simulink model "Controller_PID"  (Simulink 8.9)
settings: Solver=ode1  StartTime=0.0  StopTime=5.12  FixedStep=0.001  RelTol=1e-3
values from neighbouring files (symbols this model uses):
  Acommands = DriveCommands(:,4)-HomePosDrive(4)    [MainContourControlExp.m]    (also in MainProgress.m = Pre_commands(4,:) - HomePosCommonds(4); MainProgress02.m = output_preditionnet(4,:) - HomePosCommonds(4))
  Ccommands = DriveCommands(:,5)-HomePosDrive(5)    [MainContourControlExp.m]    (also in MainProgress.m = Pre_commands(5,:) - HomePosCommonds(5); MainProgress02.m = output_preditionnet(5,:) - HomePosCommonds(5))
  PlantADen = [1 PlantAPara.a1 PlantAPara.a0]    [MainContourControlExp.m]    (also in MainProgress.m; MainProgress02.m)
  PlantANum = [PlantAPara.b1 PlantAPara.b0]    [MainContourControlExp.m]    (also in MainProgress.m; MainProgress02.m)
  PlantCDen = [1 PlantCPara.a1 PlantCPara.a0]    [MainContourControlExp.m]    (also in MainProgress.m; MainProgress02.m)
  PlantCNum = [PlantCPara.b1 PlantCPara.b0]    [MainContourControlExp.m]    (also in MainProgress.m; MainProgress02.m)
  PlantXDen = [1 PlantXPara.a1 PlantXPara.a0]    [MainContourControlExp.m]    (also in MainProgress.m; MainProgress02.m)
  PlantXNum = [PlantXPara.b1 PlantXPara.b0]    [MainContourControlExp.m]    (also in MainProgress.m; MainProgress02.m)
  PlantYDen = [1 PlantYPara.a1 PlantYPara.a0]    [MainContourControlExp.m]    (also in MainProgress.m; MainProgress02.m)
  PlantYNum = [PlantYPara.b1 PlantYPara.b0]    [MainContourControlExp.m]    (also in MainProgress.m; MainProgress02.m)
  PlantZDen = [1 PlantZPara.a1 PlantZPara.a0]    [MainContourControlExp.m]    (also in MainProgress.m; MainProgress02.m)
  PlantZNum = [PlantZPara.b1 PlantZPara.b0]    [MainContourControlExp.m]    (also in MainProgress.m; MainProgress02.m)
  Ts = 0.001    [MainContourControlExp.m]    (also in MainProgress.m; MainProgress02.m)
  Xcommands = DriveCommands(:,1)-HomePosDrive(1)    [MainContourControlExp.m]    (also in MainProgress.m = Pre_commands(1,:) - HomePosCommonds(1); MainProgress02.m = output_preditionnet(1,:) - HomePosCommonds(1))
  Ycommands = DriveCommands(:,2)-HomePosDrive(2)    [MainContourControlExp.m]    (also in MainProgress.m = Pre_commands(2,:) - HomePosCommonds(2); MainProgress02.m = output_preditionnet(2,:) - HomePosCommonds(2))
  Zcommands = DriveCommands(:,3)-HomePosDrive(3)    [MainContourControlExp.m]    (also in MainProgress.m = Pre_commands(3,:) - HomePosCommonds(3); MainProgress02.m = output_preditionnet(3,:) - HomePosCommonds(3))
undefined symbols (not defined in the file or in its folder): DiscIntNeverNeededParam
libraries: powerlib_extras x10, simulink x5
settings Model: SuppressorTable=22 serialization::archive 11 0 6 0 0 0 11 0  Creator=e308  LastModifiedBy=e308
settings DataIOCC: LimitDataPoints=off  SaveFormat=Dataset  SignalLoggingSaveFormat=Dataset
settings OptimizationCC: LifeSpan=auto
settings DebuggingCC: UnderspecifiedInitializationDetection=Simplified  MergeDetectMultiDrivingBlocksExec=error  FcnCallInpInsideContextMsg=error  StateNameClashWarn=none  SFUnexpectedBacktrackingDiag=error  SFNoUnconditionalDefaultTransitionDiag=error  SFExecutionAtInitializationDiag=warning
settings HardwareCC: ProdBitPerPointer=64  ProdBitPerSizeT=64  ProdBitPerPtrDiffT=64  ProdLargestAtomicFloat=Float  ProdIntDivRoundTo=Zero  ProdEndianess=LittleEndian  ProdWordSize=64  ProdHWDeviceType=Intel->x86-64 (Windows64)
settings ModelReferenceCC: PropagateSignalLabelsOutOfModel=on
settings GRTTargetCC: TargetLangStandard=C99 (ISO)  GeneratePreprocessorConditionals=Use local settings  CombineOutputUpdateFcns=on  GRTInterface=off
settings ConfigComp: CovMetricSettings=dwe  CovHtmlReporting=off  CovSaveCumulativeToWorkspaceVar=off  CovSaveSingleToWorkspaceVar=off  CovExternalEMLEnable=on

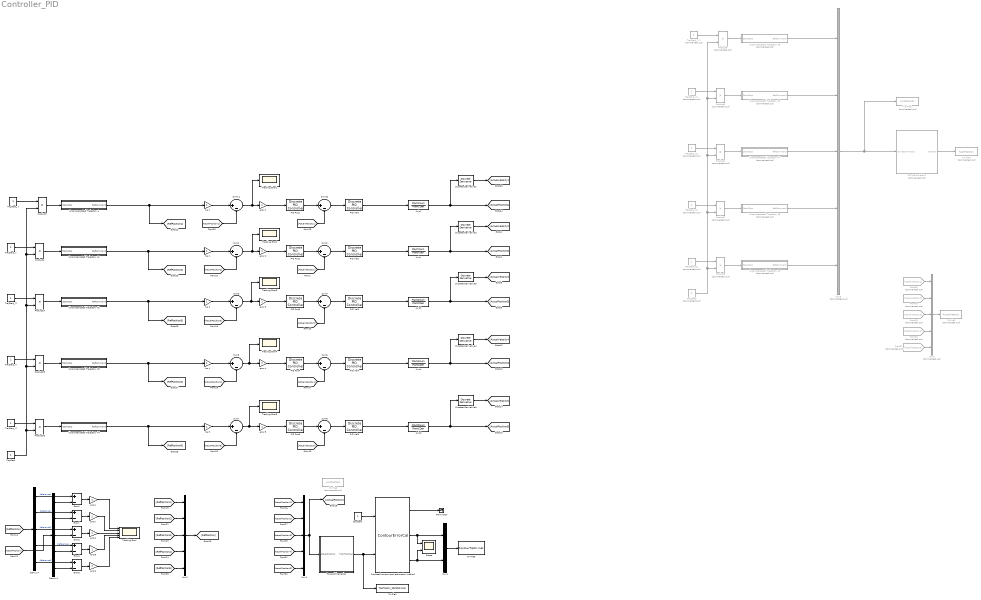
== system Controller_PID ==
  " AxisX " : DiscreteTransferFcn  Numerator=PlantXNum  Denominator=PlantXDen  SampleTime=Ts
  " AxisY" : DiscreteTransferFcn  Numerator=PlantYNum  Denominator=PlantYDen  SampleTime=Ts
  AxisA : DiscreteTransferFcn  Numerator=PlantANum  Denominator=PlantADen  SampleTime=Ts
  AxisC : DiscreteTransferFcn  Numerator=PlantCNum  Denominator=PlantCDen  SampleTime=Ts
  AxisZ : DiscreteTransferFcn  Numerator=PlantZNum  Denominator=PlantZDen  SampleTime=Ts
  Constant : Constant
  Demux1 : Demux  Outputs=5
  Demux4 : Demux  Outputs=5
  Discrete Derivative{1..5} (5 alike) : simulink/Discrete/Discrete Derivative  gainval=1.0  ICPrevScaledInput=0.0  InputProcessing=Inherited  OutMin=[]  OutMax=[]  OutDataType=fixdt(1, 16)  OutScaling=2^-10  DoSatur=off
  ErrorA : Sum  Inputs=+-
  ErrorC : Sum  Inputs=+-
  ErrorX : Sum  Inputs=+-
  ErrorY : Sum  Inputs=+-
  ErrorZ : Sum  Inputs=+-
  "ForwardKinematics " : MATLAB Function  TreatAsAtomicUnit=on
  From33 : From  Commented=on  GotoTag=ActualVelosity1
  From34 : From  Commented=on  GotoTag=ActualVelosity2
  From35 : From  Commented=on  GotoTag=ActualVelosity3
  From36 : From  Commented=on  GotoTag=ActualVelosity4
  From37 : From  Commented=on  GotoTag=ActualVelosity5
  MATLAB Function1 : MATLAB Function  Commented=on  TreatAsAtomicUnit=on
  Mux1 : Mux  Inputs=5
  Mux2 : Mux  Inputs=5
  Mux3 : Mux  Commented=on  Inputs=5
  Mux4 : Mux  Inputs=2
  Mux5 : Mux  Commented=on  Inputs=5
  PID Pos1 : powerlib_extras/Discrete  Control Blocks/Discrete PID Controller  Kp=250  Ki=0  Kd=0  TcD=0.001  Par_Limits=[1e6 -1e6]  Init=0  Ts=0.001
  PID Pos2 : powerlib_extras/Discrete  Control Blocks/Discrete PID Controller  Kp=150  Ki=0  Kd=0  TcD=0.001  Par_Limits=[1e6 -1e6]  Init=0  Ts=0.001
  PID Pos3 : powerlib_extras/Discrete  Control Blocks/Discrete PID Controller  Kp=150  Ki=0  Kd=0  TcD=0.001  Par_Limits=[1e6 -1e6]  Init=0  Ts=0.001
  PID Pos4 : powerlib_extras/Discrete  Control Blocks/Discrete PID Controller  Kp=100  Ki=0  Kd=0  TcD=0.001  Par_Limits=[1e6 -1e6]  Init=0  Ts=0.001
  PID Pos5 : powerlib_extras/Discrete  Control Blocks/Discrete PID Controller  Kp=100  Ki=0  Kd=0  TcD=0.001  Par_Limits=[1e6 -1e6]  Init=0  Ts=0.001
  PID Vel1 : powerlib_extras/Discrete  Control Blocks/Discrete PID Controller  Kp=0.01  Ki=0  Kd=0  TcD=0.001  Par_Limits=[1e6 -1e6]  Init=0  Ts=0.001
  PID Vel2 : powerlib_extras/Discrete  Control Blocks/Discrete PID Controller  Kp=0.01  Ki=0  Kd=0  TcD=0.001  Par_Limits=[1e6 -1e6]  Init=0  Ts=0.001
  PID Vel3 : powerlib_extras/Discrete  Control Blocks/Discrete PID Controller  Kp=0.01  Ki=0  Kd=0  TcD=0.001  Par_Limits=[1e6 -1e6]  Init=0  Ts=0.001
  PID Vel4 : powerlib_extras/Discrete  Control Blocks/Discrete PID Controller  Kp=0.5  Ki=0  Kd=0  TcD=0.001  Par_Limits=[1e6 -1e6]  Init=0  Ts=0.001
  PID Vel5 : powerlib_extras/Discrete  Control Blocks/Discrete PID Controller  Kp=0.5  Ki=0  Kd=0  TcD=0.001  Par_Limits=[1e6 -1e6]  Init=0  Ts=0.001
  Product{1..3,5..6} (5 alike) : Product  Commented=on  SampleTime=Ts  RndMeth=Zero
  Product{4,7,14..16} (5 alike) : Product  SampleTime=Ts  RndMeth=Zero
  Proposed contour error estimation method : S-Function  FunctionName=ContourErrorCal  Parameters=X Y Z I J K U  SFunctionDeploymentMode=off  EnableBusSupport=off
  Scope : Scope  NumInputPorts=2
  Sum{1..8,11..12} (10 alike) : Sum  Inputs=|+-
  Terminator : Terminator
  To File1 : ToFile  Filename=ToolTipOri_DNNPID.mat  MatrixName=Proposed
  To File2 : ToFile  Commented=on  Filename=ActualVelocity  MatrixName=ActualVel
  To File3 : ToFile  Commented=on  Filename=AxisPosition  MatrixName=Reference
  To File4 : ToFile  Commented=on  Filename=TaskPosition  MatrixName=ActualPos
  To File5 : ToFile  Filename=ContourTipOri.mat  MatrixName=Proposed
  To File6 : ToFile  Commented=on  Filename=AxisPosition  MatrixName=Reference
  Tracking Erro2 : Scope
  "Tracking Error " : Scope  NumInputPorts=5
  Tracking Error{1,3..5} (4 alike) : Scope
  TrajStart : Constant
  TrajStart1 : Constant  Commented=on
  TrajStart_ A : Constant
  TrajStart_ A1 : Constant  Commented=on
  TrajStart_ C : Constant
  TrajStart_ C1 : Constant  Commented=on
  "TrajStart_ X " : Constant
  TrajStart_ X 1 : Constant  Commented=on
  TrajStart_ Y : Constant
  TrajStart_ Y1 : Constant  Commented=on
  TrajStart_ Z : Constant
  TrajStart_ Z1 : Constant  Commented=on
  Uncompensated Trajectory A : Subsystem
  Uncompensated Trajectory A1 : Subsystem
  Uncompensated Trajectory A2 : Subsystem
  Uncompensated Trajectory A3 : Subsystem
  Uncompensated Trajectory A4 : Subsystem
  Uncompensated Trajectory A5 : Subsystem  Commented=on
  Uncompensated Trajectory A6 : Subsystem  Commented=on
  Uncompensated Trajectory A7 : Subsystem  Commented=on
  Uncompensated Trajectory A8 : Subsystem  Commented=on
  Uncompensated Trajectory A9 : Subsystem  Commented=on
  error {1..5} (5 alike) : Gain
  errora : Gain  SampleTime=0.001
  errorc : Gain  SampleTime=0.001
  errorx : Gain  SampleTime=0.001
  errory : Gain  SampleTime=0.001
  errorz : Gain  SampleTime=0.001
  tra {1..5} (5 alike) : Gain
  wires:
  [RefPosition5] -> Mux2/5
  [RefPosition4] -> Mux2/4
  [RefPosition3] -> Mux2/3
  Sum11/1 -> Tracking Error1/1, error 1/1
  [RefPosition2] -> Mux2/2
  From33/1 -> Mux3/1
  Discrete Derivative5/1 -> [ActualVelosity5]
  Sum3/1 -> error 3/1, Tracking Error3/1
  From36/1 -> Mux3/4
  Discrete Derivative3/1 -> [ActualVelosity3]
  Discrete Derivative2/1 -> [ActualVelosity2]
  [ActualVelosity3] -> Sum4/2
  error 4/1 -> PID Pos4/1
  Product2/1 -> Uncompensated Trajectory A8/1(Start-Stop)
  Demux4/5 -> ErrorC/1  "ReferenceC"
  [ActualPosition1] -> Sum11/2
  " AxisY"/1 -> Discrete Derivative2/1, [ActualPosition2]
  Uncompensated Trajectory A9/1(RefCommand) -> Mux5/5
  Demux4/3 -> ErrorZ/1  "ReferenceZ"
  Discrete Derivative1/1 -> [ActualVelosity1]
  tra 5/1 -> Sum7/1
  Sum7/1 -> error 5/1, Tracking Error5/1
  [ActualVelosity5] -> Sum8/2
  errorz/1 -> "Tracking Error "/3
  Uncompensated Trajectory A1/1(RefCommand) -> [RefPosition2], tra 2/1
  PID Vel4/1 -> AxisA/1
  Sum5/1 -> error 4/1, Tracking Error4/1
  PID Pos1/1 -> Sum12/1
  Demux4/1 -> ErrorX/1  "ReferenceX"
  PID Pos5/1 -> Sum8/1
  MATLAB Function1/1(TipOrien) -> To File4/1
  tra 4/1 -> Sum5/1
  [RefPosition1] -> Mux2/1
  [ActualVelosity4] -> Sum6/2
  errorx/1 -> "Tracking Error "/1
  [ActualPosition] -> Demux1/1
  Sum12/1 -> PID Vel1/1
  Uncompensated Trajectory A5/1(RefCommand) -> Mux5/1
  Product15/1 -> Uncompensated Trajectory A3/1(Start-Stop)
  errorc/1 -> "Tracking Error "/5
  Proposed contour error estimation method/1 -> Terminator/1
  Demux1/2 -> ErrorY/2
  Sum4/1 -> PID Vel3/1
  errora/1 -> "Tracking Error "/4
  PID Pos4/1 -> Sum6/1
  Demux1/5 -> ErrorC/2
  TrajStart_ Y/1 -> Product4/1
  TrajStart/1 -> Product16/2, Product15/2, Product14/2, Product7/2, Product4/2
  tra 2/1 -> Sum1/1
  [ActualVelosity2] -> Sum2/2
  ErrorC/1 -> errorc/1
  Product16/1 -> Uncompensated Trajectory A4/1(Start-Stop)
  AxisZ/1 -> Discrete Derivative3/1, [ActualPosition3]
  "ForwardKinematics "/1(ToolTipOrien) -> To File1/1, Proposed contour error estimation method/2
  TrajStart_ X 1/1 -> Product6/1
  Uncompensated Trajectory A3/1(RefCommand) -> [RefPosition4], tra 4/1
  Product6/1 -> Uncompensated Trajectory A5/1(Start-Stop)
  TrajStart_ Z/1 -> Product14/1
  Uncompensated Trajectory A8/1(RefCommand) -> Mux5/4
  tra 3/1 -> Sum3/1
  Product4/1 -> Uncompensated Trajectory A1/1(Start-Stop)
  AxisA/1 -> Discrete Derivative4/1, [ActualPosition4]
  PID Pos2/1 -> Sum2/1
  TrajStart_ C1/1 -> Product3/1
  ErrorZ/1 -> errorz/1
  TrajStart_ C/1 -> Product16/1
  TrajStart_ A/1 -> Product15/1
  Sum2/1 -> PID Vel2/1
  PID Pos3/1 -> Sum4/1
  Demux4/2 -> ErrorY/1  "ReferenceY"
  error 2/1 -> PID Pos2/1
  Uncompensated Trajectory A/1(RefCommand) -> [RefPosition1], tra 1/1
  " AxisX "/1 -> Discrete Derivative1/1, [ActualPosition1]
  [ActualPosition2] -> Mux1/2
  ErrorY/1 -> errory/1
  tra 1/1 -> Sum11/1
  [ActualVelosity1] -> Sum12/2
  Uncompensated Trajectory A4/1(RefCommand) -> [RefPosition5], tra 5/1
  [ActualPosition4] -> Sum5/2
  [ActualPosition3] -> Sum3/2
  From35/1 -> Mux3/3
  [ActualPosition2] -> Sum1/2
  AxisC/1 -> Discrete Derivative5/1, [ActualPosition5]
  [ActualPosition5] -> Sum7/2
  TrajStart_ Z1/1 -> Product1/1
  Demux1/4 -> ErrorA/2
  Uncompensated Trajectory A2/1(RefCommand) -> [RefPosition3], tra 3/1
  Product1/1 -> Uncompensated Trajectory A7/1(Start-Stop)
  "TrajStart_ X "/1 -> Product7/1
  [ActualPosition3] -> Mux1/3
  PID Vel5/1 -> AxisC/1
  ErrorX/1 -> errorx/1
  Mux3/1 -> To File2/1
  PID Vel1/1 -> " AxisX "/1
  [RefPosition] -> Demux4/1
  Demux1/1 -> ErrorX/2
  error 3/1 -> PID Pos3/1
  PID Vel2/1 -> " AxisY"/1
  Product14/1 -> Uncompensated Trajectory A2/1(Start-Stop)
  Product3/1 -> Uncompensated Trajectory A9/1(Start-Stop)
  PID Vel3/1 -> AxisZ/1
  From34/1 -> Mux3/2
  Product5/1 -> Uncompensated Trajectory A6/1(Start-Stop)
  Demux1/3 -> ErrorZ/2
  [ActualPosition1] -> Mux1/1
  TrajStart_ Y1/1 -> Product5/1
  TrajStart_ A1/1 -> Product2/1
  Demux4/4 -> ErrorA/1  "ReferenceA"
  From37/1 -> Mux3/5
  error 5/1 -> PID Pos5/1
  [ActualPosition4] -> Mux1/4
  Mux1/1 -> [ActualPosition], "ForwardKinematics "/1(ActualPosition)
  Product7/1 -> Uncompensated Trajectory A/1(Start-Stop)
  Uncompensated Trajectory A6/1(RefCommand) -> Mux5/2
  Mux2/1 -> [RefPosition]
  Sum6/1 -> PID Vel4/1
  Sum1/1 -> Tracking Erro2/1, error 2/1
  Proposed contour error estimation method/2 -> Mux4/1, Scope/1
  Constant/1 -> Proposed contour error estimation method/1
  Sum8/1 -> PID Vel5/1
  Discrete Derivative4/1 -> [ActualVelosity4]
  errory/1 -> "Tracking Error "/2
  Mux5/1 -> MATLAB Function1/1(DriveCommands), To File6/1
  Uncompensated Trajectory A7/1(RefCommand) -> Mux5/3
  Proposed contour error estimation method/3 -> Mux4/2, Scope/2
  [ActualPosition5] -> Mux1/5
  TrajStart1/1 -> Product3/2, Product2/2, Product1/2, Product6/2, Product5/2
  Mux4/1 -> To File5/1
  error 1/1 -> PID Pos1/1
  ErrorA/1 -> errora/1

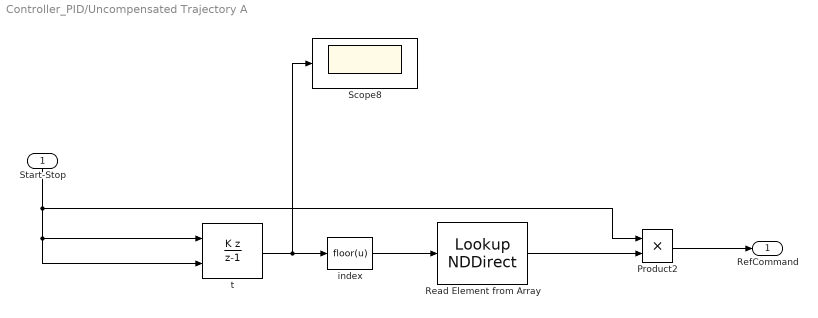
== system Controller_PID/Uncompensated Trajectory A ==
  Start-Stop : Inport
  Product2 : Product  RndMeth=Zero
  Read Element from Array : LookupNDDirect  NumberOfTableDimensions=1  Table=Xcommands
  Scope8 : Scope
  index : Fcn  Expr=floor(u)
  t : DiscreteIntegrator  IntegratorMethod=Accumulation: Backward Euler  ExternalReset=rising  SampleTime=Ts  ICPrevOutput=DiscIntNeverNeededParam  ICPrevScaledInput=DiscIntNeverNeededParam
  RefCommand : Outport
  wires:
  Read Element from Array/1 -> Product2/2
  t/1 -> Scope8/1, index/1
  Product2/1 -> RefCommand/1
  Start-Stop/1 -> Product2/1, t/1, t/2
  index/1 -> Read Element from Array/1

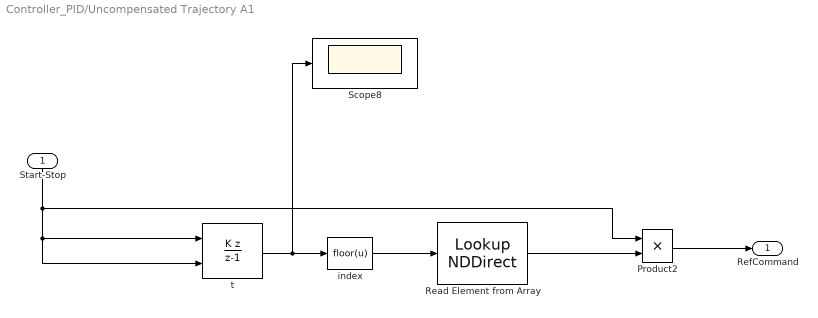
== system Controller_PID/Uncompensated Trajectory A1 ==
  Start-Stop : Inport
  Product2 : Product  RndMeth=Zero
  Read Element from Array : LookupNDDirect  NumberOfTableDimensions=1  Table=Ycommands
  Scope8 : Scope
  index : Fcn  Expr=floor(u)
  t : DiscreteIntegrator  IntegratorMethod=Accumulation: Backward Euler  ExternalReset=rising  SampleTime=Ts  ICPrevOutput=DiscIntNeverNeededParam  ICPrevScaledInput=DiscIntNeverNeededParam
  RefCommand : Outport
  wires:
  index/1 -> Read Element from Array/1
  Start-Stop/1 -> t/2, t/1, Product2/1
  Product2/1 -> RefCommand/1
  t/1 -> index/1, Scope8/1
  Read Element from Array/1 -> Product2/2

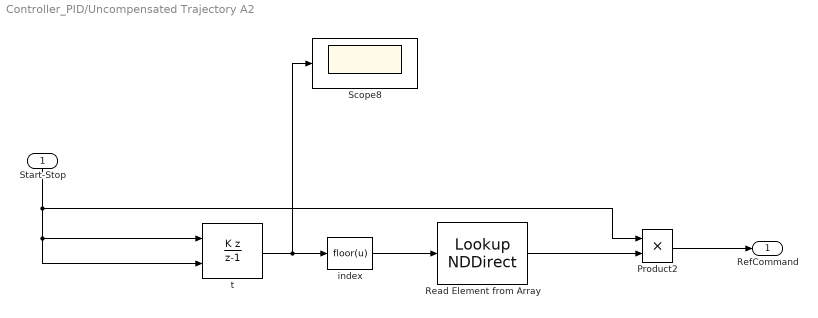
== system Controller_PID/Uncompensated Trajectory A2 ==
  Start-Stop : Inport
  Product2 : Product  RndMeth=Zero
  Read Element from Array : LookupNDDirect  NumberOfTableDimensions=1  Table=Zcommands
  Scope8 : Scope
  index : Fcn  Expr=floor(u)
  t : DiscreteIntegrator  IntegratorMethod=Accumulation: Backward Euler  ExternalReset=rising  SampleTime=Ts  ICPrevOutput=DiscIntNeverNeededParam  ICPrevScaledInput=DiscIntNeverNeededParam
  RefCommand : Outport
  wires:
  Read Element from Array/1 -> Product2/2
  t/1 -> Scope8/1, index/1
  Product2/1 -> RefCommand/1
  Start-Stop/1 -> Product2/1, t/1, t/2
  index/1 -> Read Element from Array/1

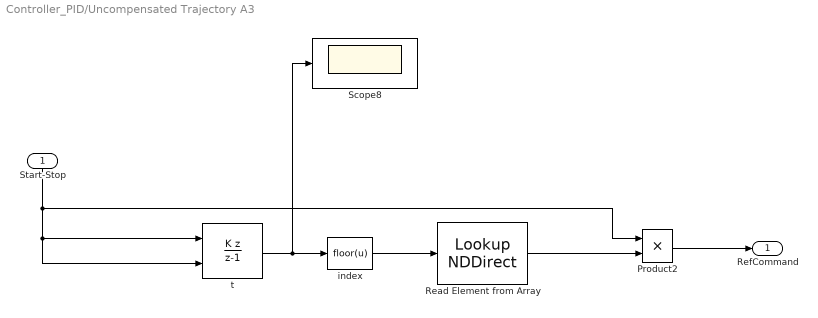
== system Controller_PID/Uncompensated Trajectory A3 ==
  Start-Stop : Inport
  Product2 : Product  RndMeth=Zero
  Read Element from Array : LookupNDDirect  NumberOfTableDimensions=1  Table=Acommands
  Scope8 : Scope
  index : Fcn  Expr=floor(u)
  t : DiscreteIntegrator  IntegratorMethod=Accumulation: Backward Euler  ExternalReset=rising  SampleTime=Ts  ICPrevOutput=DiscIntNeverNeededParam  ICPrevScaledInput=DiscIntNeverNeededParam
  RefCommand : Outport
  wires:
  index/1 -> Read Element from Array/1
  Start-Stop/1 -> t/2, t/1, Product2/1
  Product2/1 -> RefCommand/1
  t/1 -> index/1, Scope8/1
  Read Element from Array/1 -> Product2/2

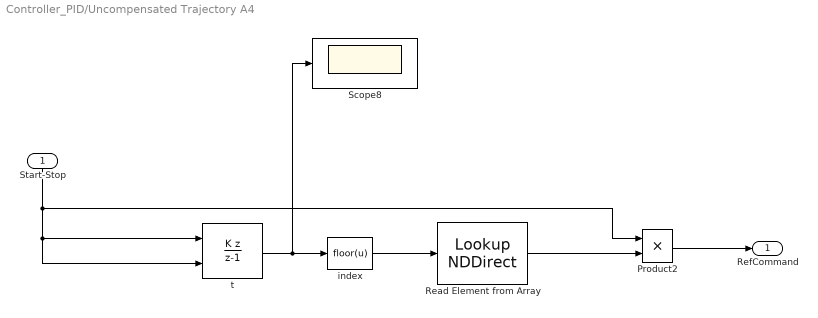
== system Controller_PID/Uncompensated Trajectory A4 ==
  Start-Stop : Inport
  Product2 : Product  RndMeth=Zero
  Read Element from Array : LookupNDDirect  NumberOfTableDimensions=1  Table=Ccommands
  Scope8 : Scope
  index : Fcn  Expr=floor(u)
  t : DiscreteIntegrator  IntegratorMethod=Accumulation: Backward Euler  ExternalReset=rising  SampleTime=Ts  ICPrevOutput=DiscIntNeverNeededParam  ICPrevScaledInput=DiscIntNeverNeededParam
  RefCommand : Outport
  wires:
  Read Element from Array/1 -> Product2/2
  t/1 -> Scope8/1, index/1
  Product2/1 -> RefCommand/1
  Start-Stop/1 -> Product2/1, t/1, t/2
  index/1 -> Read Element from Array/1

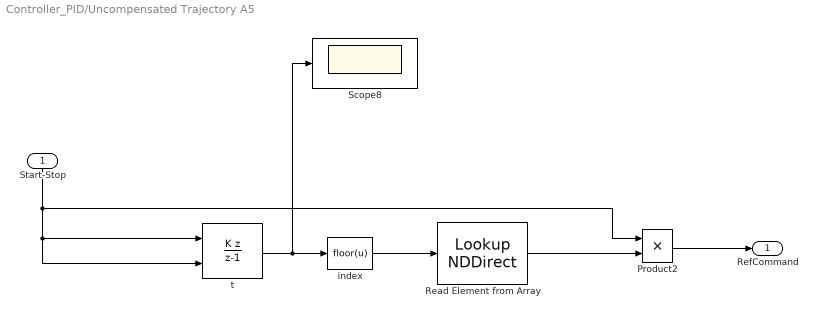
== system Controller_PID/Uncompensated Trajectory A5 ==
  Start-Stop : Inport
  Product2 : Product  RndMeth=Zero
  Read Element from Array : LookupNDDirect  NumberOfTableDimensions=1  Table=Xcommands
  Scope8 : Scope
  index : Fcn  Expr=floor(u)
  t : DiscreteIntegrator  IntegratorMethod=Accumulation: Backward Euler  ExternalReset=rising  SampleTime=Ts  ICPrevOutput=DiscIntNeverNeededParam  ICPrevScaledInput=DiscIntNeverNeededParam
  RefCommand : Outport
  wires:
  Read Element from Array/1 -> Product2/2
  t/1 -> Scope8/1, index/1
  Product2/1 -> RefCommand/1
  Start-Stop/1 -> Product2/1, t/1, t/2
  index/1 -> Read Element from Array/1

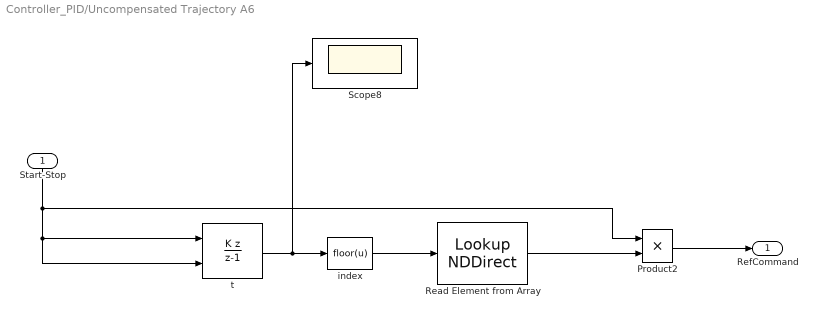
== system Controller_PID/Uncompensated Trajectory A6 ==
  Start-Stop : Inport
  Product2 : Product  RndMeth=Zero
  Read Element from Array : LookupNDDirect  NumberOfTableDimensions=1  Table=Ycommands
  Scope8 : Scope
  index : Fcn  Expr=floor(u)
  t : DiscreteIntegrator  IntegratorMethod=Accumulation: Backward Euler  ExternalReset=rising  SampleTime=Ts  ICPrevOutput=DiscIntNeverNeededParam  ICPrevScaledInput=DiscIntNeverNeededParam
  RefCommand : Outport
  wires:
  index/1 -> Read Element from Array/1
  Start-Stop/1 -> t/2, t/1, Product2/1
  Product2/1 -> RefCommand/1
  t/1 -> index/1, Scope8/1
  Read Element from Array/1 -> Product2/2

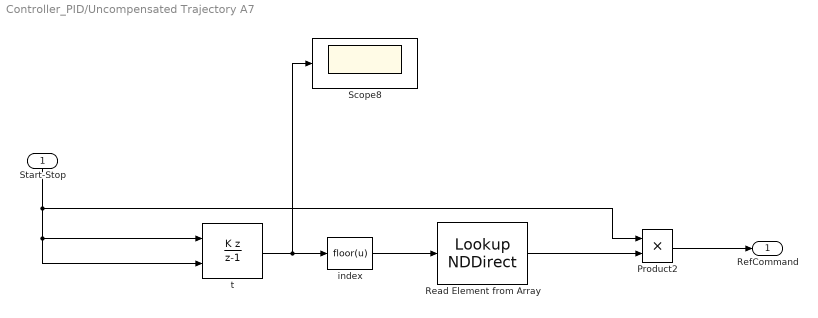
== system Controller_PID/Uncompensated Trajectory A7 ==
  Start-Stop : Inport
  Product2 : Product  RndMeth=Zero
  Read Element from Array : LookupNDDirect  NumberOfTableDimensions=1  Table=Zcommands
  Scope8 : Scope
  index : Fcn  Expr=floor(u)
  t : DiscreteIntegrator  IntegratorMethod=Accumulation: Backward Euler  ExternalReset=rising  SampleTime=Ts  ICPrevOutput=DiscIntNeverNeededParam  ICPrevScaledInput=DiscIntNeverNeededParam
  RefCommand : Outport
  wires:
  Read Element from Array/1 -> Product2/2
  t/1 -> Scope8/1, index/1
  Product2/1 -> RefCommand/1
  Start-Stop/1 -> Product2/1, t/1, t/2
  index/1 -> Read Element from Array/1

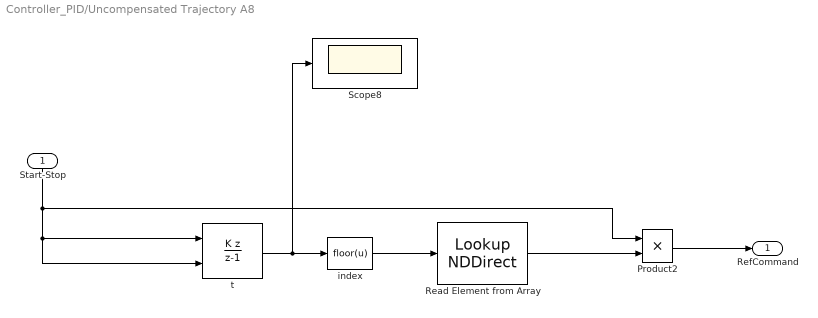
== system Controller_PID/Uncompensated Trajectory A8 ==
  Start-Stop : Inport
  Product2 : Product  RndMeth=Zero
  Read Element from Array : LookupNDDirect  NumberOfTableDimensions=1  Table=Acommands
  Scope8 : Scope
  index : Fcn  Expr=floor(u)
  t : DiscreteIntegrator  IntegratorMethod=Accumulation: Backward Euler  ExternalReset=rising  SampleTime=Ts  ICPrevOutput=DiscIntNeverNeededParam  ICPrevScaledInput=DiscIntNeverNeededParam
  RefCommand : Outport
  wires:
  index/1 -> Read Element from Array/1
  Start-Stop/1 -> t/2, t/1, Product2/1
  Product2/1 -> RefCommand/1
  t/1 -> index/1, Scope8/1
  Read Element from Array/1 -> Product2/2

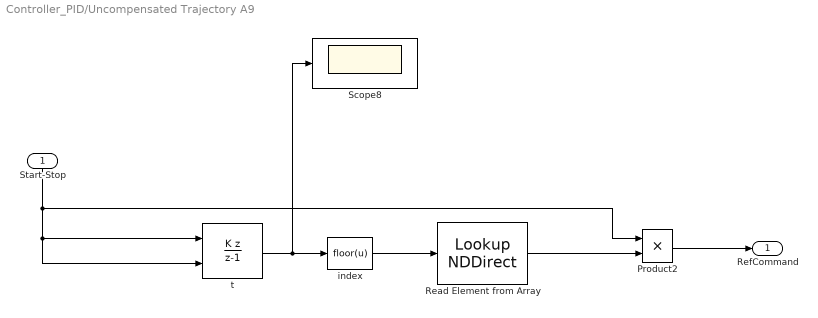
== system Controller_PID/Uncompensated Trajectory A9 ==
  Start-Stop : Inport
  Product2 : Product  RndMeth=Zero
  Read Element from Array : LookupNDDirect  NumberOfTableDimensions=1  Table=Ccommands
  Scope8 : Scope
  index : Fcn  Expr=floor(u)
  t : DiscreteIntegrator  IntegratorMethod=Accumulation: Backward Euler  ExternalReset=rising  SampleTime=Ts  ICPrevOutput=DiscIntNeverNeededParam  ICPrevScaledInput=DiscIntNeverNeededParam
  RefCommand : Outport
  wires:
  Read Element from Array/1 -> Product2/2
  t/1 -> Scope8/1, index/1
  Product2/1 -> RefCommand/1
  Start-Stop/1 -> Product2/1, t/1, t/2
  index/1 -> Read Element from Array/1

== matlab function MATLAB Function1 ==
  data: DriveCommands input double; TipOrien output double
function TipOrien = ForwardKinematics(DriveCommands)

Lacy = 0;
Lacz = 41;

HomePosDrive=[113.232633012931,18.4363460319427,0.239716132104988,0.686766850928449,-0.169983380596482];
% HomePosDrive=[0,0,0,0,0];

X = DriveCommands(1)+HomePosDrive(1);
Y = DriveCommands(2)+HomePosDrive(2);
Z = DriveCommands(3)+HomePosDrive(3);
A = DriveCommands(4)+HomePosDrive(4);
C = DriveCommands(5)+HomePosDrive(5);


Oi = sin(A)*sin(C);
Oj = sin(A)*cos(C);
Ok = cos(A);
Px = cos(C)*X+cos(A)*sin(C)*Y+sin(A)*sin(C)*Z-cos(A)*sin(C)*Lacy-sin(A)*sin(C)*Lacz;
Py = -sin(C)*X+cos(A)*cos(C)*Y+sin(A)*cos(C)*Z+(1-cos(A)*cos(C))*Lacy-sin(A)*cos(C)*Lacz;
Pz = -sin(A)*Y+cos(A)*Z+sin(A)*Lacy+(1-cos(A))*Lacz;

TipOrien = [Px Py Pz Oi Oj Ok]';

== matlab function ForwardKinematics  ==
  data: ActualPosition input double; ToolTipOrien output double; HomePosCommonds parameter double

function ToolTipOrien=ForwardKinematics(ActualPosition,HomePosCommonds)

Lacy = 0;
Lacz = 41;

X = ActualPosition(1)+HomePosCommonds(1);
Y = ActualPosition(2)+HomePosCommonds(2);
Z = ActualPosition(3)+HomePosCommonds(3);
A = ActualPosition(4)+HomePosCommonds(4);
C = ActualPosition(5)+HomePosCommonds(5);

Px = cos(C)*X+cos(A)*sin(C)*Y+sin(A)*sin(C)*Z-cos(A)*sin(C)*Lacy-sin(A)*sin(C)*Lacz;
Py = -sin(C)*X+cos(A)*cos(C)*Y+sin(A)*cos(C)*Z+(1-cos(A)*cos(C))*Lacy-sin(A)*cos(C)*Lacz;
Pz = -sin(A)*Y+cos(A)*Z+sin(A)*Lacy+(1-cos(A))*Lacz;

Oi = sin(A)*sin(C);
Oj = sin(A)*cos(C);
Ok = cos(A);

ToolTipOrien=[Px Py Pz Oi Oj Ok A C]';
end
